simulink model "RT_poles_epsilon"  (Simulink 8.1)
settings: Solver=ode45  StartTime=0.0  StopTime=10.0  RelTol=1e-3
settings Model: Creator=mainster  LastModifiedBy=mainster
settings DataIOCC: SignalLoggingSaveFormat=Dataset
settings OptimizationCC: ExpressionDepthLimit=128
settings DebuggingCC: SolverPrmCheckMsg=none  FcnCallInpInsideContextMsg=EnableAllAsError
settings GRTTargetCC: CombineOutputUpdateFcns=on  GRTInterface=off

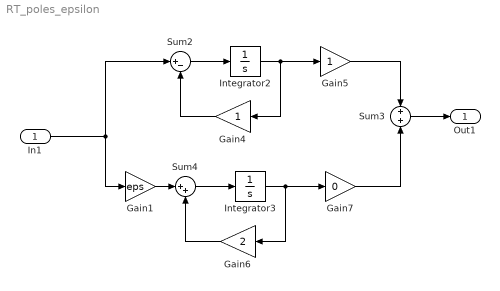
== system RT_poles_epsilon ==
  In1 : Inport
  Gain1 : Gain  Gain=eps
  Gain4 : Gain
  Gain5 : Gain
  Gain6 : Gain  Gain=2
  Gain7 : Gain  Gain=0
  Integrator2 : Integrator
  Integrator3 : Integrator
  Sum2 : Sum  Inputs=|+-
  Sum3 : Sum  Inputs=+|+
  Sum4 : Sum  Inputs=|++
  Out1 : Outport
  wires:
  Sum2/1 -> Integrator2/1
  Integrator2/1 -> Gain5/1, Gain4/1
  In1/1 -> Sum2/1, Gain1/1
  Gain4/1 -> Sum2/2
  Gain5/1 -> Sum3/1
  Sum4/1 -> Integrator3/1
  Integrator3/1 -> Gain7/1, Gain6/1
  Gain6/1 -> Sum4/2
  Gain7/1 -> Sum3/2
  Sum3/1 -> Out1/1
  Gain1/1 -> Sum4/1
